simulink model "outer_axe"  (R2021a)
settings: Solver=VariableStepAuto  StartTime=0.0  StopTime=10.0  RelTol=1e-3
settings Model: Creator=user  LastModifiedBy=user

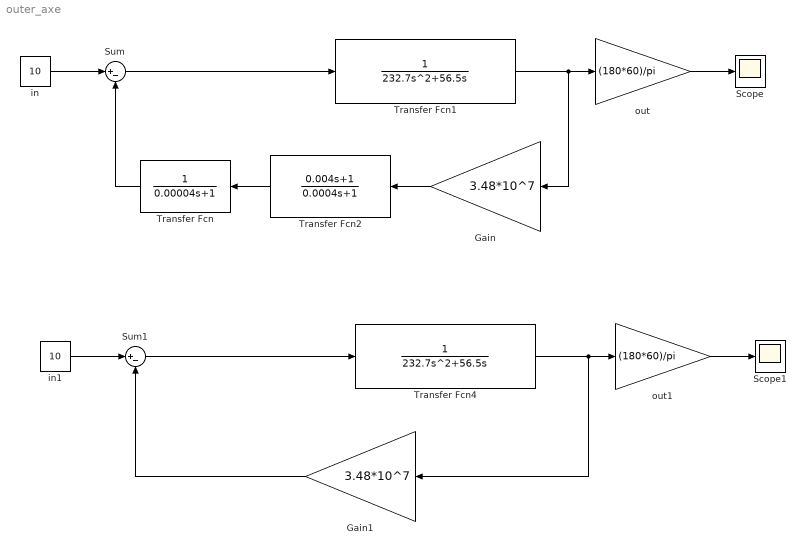
== system outer_axe ==
  Gain : Gain  Gain=3.48*10^7
  Gain1 : Gain  Gain=3.48*10^7
  Scope : Scope
  Scope1 : Scope
  Sum : Sum  Inputs=|+-
  Sum1 : Sum  Inputs=|+-
  Transfer Fcn : TransferFcn  Denominator=[0.00004 1]
  Transfer Fcn1 : TransferFcn  Denominator=[232.7 56.5 0]
  Transfer Fcn2 : TransferFcn  Numerator=[0.004 1]  Denominator=[0.0004 1]
  Transfer Fcn4 : TransferFcn  Denominator=[232.7 56.5 0]
  in : Constant  Value=10  SampleTime=1
  in1 : Constant  Value=10  SampleTime=1
  out : Gain  Gain=(180*60)/pi
  out1 : Gain  Gain=(180*60)/pi
  wires:
  Transfer Fcn/1 -> Sum/2
  in/1 -> Sum/1
  out/1 -> Scope/1
  Transfer Fcn2/1 -> Transfer Fcn/1
  Sum/1 -> Transfer Fcn1/1
  Gain/1 -> Transfer Fcn2/1
  Transfer Fcn1/1 -> Gain/1, out/1
  Transfer Fcn4/1 -> Gain1/1, out1/1
  Sum1/1 -> Transfer Fcn4/1
  out1/1 -> Scope1/1
  in1/1 -> Sum1/1
  Gain1/1 -> Sum1/2
